simulink model "Bus_Selector"  (R2014a)
settings: Solver=FixedStepDiscrete  StartTime=0.0  StopTime=10.0  FixedStep=0.1  RelTol=1e-3
settings Model: BufferReuse=off  Creator=kohei-y  LastModifiedBy=ts1413
settings OptimizationCC: BlockReduction=off  OptimizeBlockIOStorage=off  BufferReuse=off  GlobalBufferReuse=off  ExpressionFolding=off  LocalBlockOutputs=off  OptimizeModelRefInitCode=on  LifeSpan=1
settings RTWCC: SystemTargetFile=ert.tlc  GenCodeOnly=on  TemplateMakefile=ert_default_tmf  Description=Embedded Coder  ProcessScript=ert_make_rtw_hook  IncludeHyperlinkInReport=on
settings CodeAppCC: IgnoreCustomStorageClasses=off
settings ERTTargetCC: ParMdlRefBuildCompliant=on  CompOptLevelCompliant=on  ConcurrentExecutionCompliant=on  ERTFirstTimeCompliant=on  ModelStepFunctionPrototypeControlCompliant=on  CPPClassGenCompliant=on  InlinedParameterPlacement=Hierarchical  ERTCustomFileTemplate=example_file_process.tlc

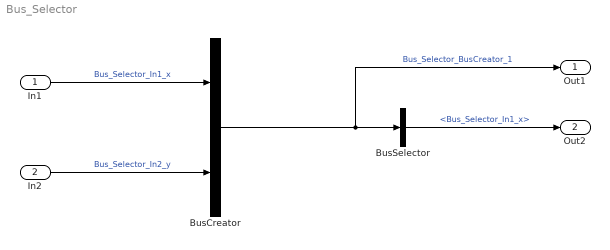
== system Bus_Selector ==
  In1 : Inport
  In2 : Inport  Port=2
  BusCreator : BusCreator  Inputs=2
  BusSelector : BusSelector  OutputSignals=Bus_Selector_In1_x
  Out1 : Outport
  Out2 : Outport  Port=2
  wires:
  In1/1 -> BusCreator/1  "Bus_Selector_In1_x"
  In2/1 -> BusCreator/2  "Bus_Selector_In2_y"
  BusCreator/1 -> BusSelector/1, Out1/1  "Bus_Selector_BusCreator_1"
  BusSelector/1 -> Out2/1  "<Bus_Selector_In1_x>"
